simulink model "mpu6050_serial_lpf"  (R2023b)
settings: Solver=VariableStepAuto  StartTime=0.0  StopTime=inf  FixedStep=0.01  RelTol=1e-3
settings Model: Creator=mly  LastModifiedBy=mly

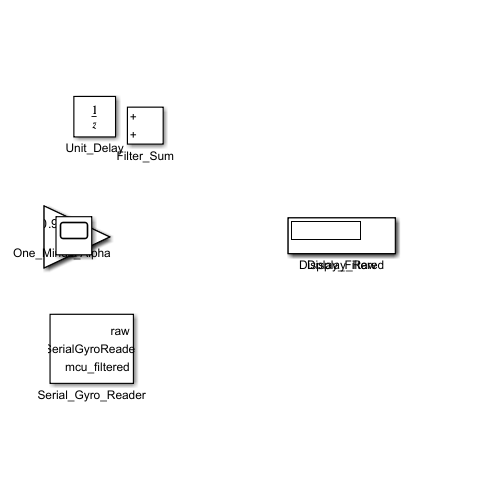
[thumbnail: Simulink's stored preview of the top-level diagram]
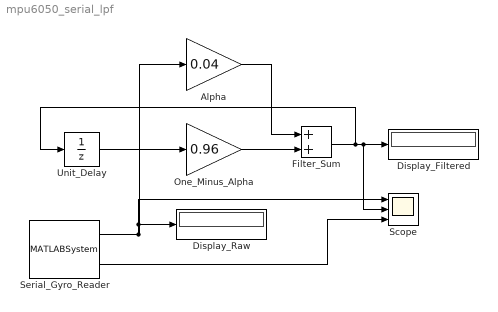
== system mpu6050_serial_lpf ==
  Alpha : Gain  Gain=0.04
  Display_Filtered : Display
  Display_Raw : Display
  Filter_Sum : Sum
  One_Minus_Alpha : Gain  Gain=0.96
  Scope : Scope  NumInputPorts=3
  Serial_Gyro_Reader : MATLABSystem  System=SerialGyroReader  COMPort=COM3  BaudRate=115200  SimulateUsing=Code generation
      mask Type: SerialGyroReader
      mask Display:
      | disp('SerialGyroReader');
      | port_label('output',1,'raw');
      | port_label('output',2,'mcu_filtered');
  Unit_Delay : UnitDelay  SampleTime=0.01  HasFrameUpgradeWarning=on
  wires:
  Alpha/1 -> Filter_Sum/1
  Serial_Gyro_Reader/2 -> Scope/3
  Unit_Delay/1 -> One_Minus_Alpha/1
  Serial_Gyro_Reader/1 -> Scope/1, Display_Raw/1, Alpha/1
  One_Minus_Alpha/1 -> Filter_Sum/2
  Filter_Sum/1 -> Scope/2, Display_Filtered/1, Unit_Delay/1
